simulink library "SUB_L4_Task_10ms_SUB_STEERCTRL"  (R2018a)
settings: Solver=VariableStepAuto  StartTime=0.0  StopTime=10.0  RelTol=1e-3
undefined symbols (not defined in the file or in its folder): Curvature_FF_Gain, DiscIntNeverNeededParam, Lateral_Control_Curvature_Limit, Lateral_Control_D, Lateral_Control_Error_Limit, Lateral_Control_Error_Rate_Limit, Lateral_Control_I, Lateral_Control_P, Lateral_Control_Rate_Limit_APV, Lateral_Control_YawRate_Limit, ptc_matlab_lib, REAX_OFFSET_APV, STANLEY_GAIN_APV, UndersteerCorection, Yaw_Rate_FF_Gain
libraries: EmE_MBD_Blockset x16, simulink x9, PTC_MBDS_LIB x3
settings Model: Creator=Chris.Balton  LastModifiedBy=Gavin.Coelho

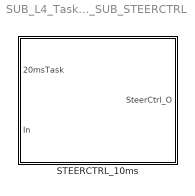
== system SUB_L4_Task_10ms_SUB_STEERCTRL ==
  STEERCTRL_10ms : Subsystem

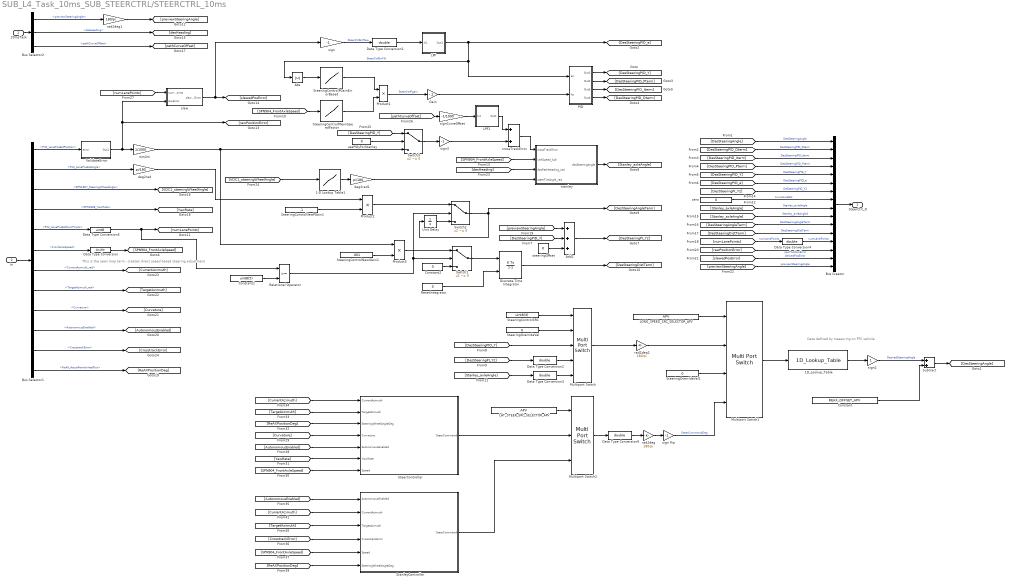
== system SUB_L4_Task_10ms_SUB_STEERCTRL/STEERCTRL_10ms ==
  note: This is the open loop term - creates direct speed based steering adjustment
  note: Data defined by measuring on PTC vehicle
  20msTask : Inport
  In : Inport  Port=2
  1-D Lookup Table1 : Lookup_n-D  NumberOfTableDimensions=1  BreakpointsForDimension1=|  Table=|  InternalRulePriority=Speed  RndMeth=Simplest  InputSameDT=on
      BreakpointsForDimension1=|
      | [-800
      | -700
      | -600
      | -500
      | -400
      | -300
      | -200
      | -100
      | 0
      | 100
      | 200
      | 300
      | 400
      | 500
      | 600
      | 700
      | 800
      | ]
      Table=|
      | [-46
      | -39.5
      | -33.5
      | -27
      | -21.5
      | -16
      | -10
      | -4.5
      | 0
      | 5.5
      | 11
      | 16
      | 21.5
      | 26
      | 31
      | 33
      | 33
      | ]
  1D_Lookup_Table : PTC_MBDS_LIB/Extras/Lookup Tables/1D_Lookup_Table  ParameterObjectName=STEERCTRL_WHEEL_ANGLE_DATA_MPV  InterpolationMethod=Linear  PTC_MBDS_BlockVersion=5.41  PTC_BlockType=PTC_MBDS_1D_Lookup_Table
      settings: SourceProductName=PACCAR Technical Center MBDS Library
      settings: AttributesFormatString=|
      | X Axis: STEERCTRL_WHEEL_ANGLE_STEP_MPV (deg)
      | Y Axis: STEERCTRL_WHEEL_ANGLE_DATA_MPV (deg)
      | Interpolation Method: Linear
  Abs : Abs
  Add2 : Sum  Inputs=+++
  Bus Creator : BusCreator  Inputs=16
  Bus Selector1 : BusSelector  OutputSignals=CAN.PX2_Lane.LanePosEst.PX2_LanePosEstPosition,CAN.PX2_Lane.LanePosEst.PX2_LanePosEstAngle,CAN.VDC2_0B.SPN1807_SteeringWheelAngle,CAN.VDC2_0B.SPN1808_YawRate,CAN.PX2_Lane.LanePosEst.PX2_LanePosEstNumPoints,CAN.EBC2_0B.FrontAxleSpeed,PIC_Bus.CurrentAzimuth_rad,PIC_Bus.TargetAzimuth_rad,PIC_Bus.Curvature,AutonomousState.AutonomousEnabled,PIC_Bus.CrosstrackError,CAN.ReAX.ReAX_ActualHandwheelPos
  Bus Selector2 : BusSelector  OutputSignals=mapping.previewSteeringAngle,mapping.desHeading,mapping.pathCurveOffset
  Constant : Constant  Value=REAX_OFFSET_APV
  Constant1 : Constant  Value=uint8(5)
  Constant2 : Constant  Value=0
  Data Type Conversion{,1..4,6} (6 alike) : DataTypeConversion  OutDataTypeStr=double
  Data Type Conversion5 : DataTypeConversion  OutDataTypeStr=uint8
  Discrete-Time Integrator : DiscreteIntegrator  ExternalReset=level  SampleTime=.01  LimitOutput=on  UpperSaturationLimit=1000  LowerSaturationLimit=-1000  ICPrevOutput=DiscIntNeverNeededParam  ICPrevScaledInput=DiscIntNeverNeededParam
  Gain : Gain  Gain=-.2
  LAT_STEER_SRC_SELECTOR_APV : EmE_MBD_Blockset/Sources/APV  conval=LAT_STEER_SRC_SELECTOR_APV
      settings: SourceProductName=PACCAR EmE MBD Blockset
  LONG_SPEED_SRC_SELECTOR_APV : EmE_MBD_Blockset/Sources/APV  conval=LONG_SPEED_SRC_SELECTOR_APV
      settings: SourceProductName=PACCAR EmE MBD Blockset
  LPF : Subsystem
  LPF1 : Subsystem
  Multiport Switch : MultiPortSwitch  DataPortOrder=Zero-based contiguous  Inputs=4  zeroidx=on
  Multiport Switch1 : MultiPortSwitch  DataPortOrder=Specify indices  DataPortIndices={ENUM_LONG_SPEED_DEMAND_SOURCE_T.GPS_PATH,ENUM_LONG_SPEED_DEMAND_SOURCE_T.OVERRIDE,ENUM_LONG_SPEED_DEMAND_SOURCE_T.WAYPOINTS}  DiagnosticForDefault=None
  Multiport Switch2 : MultiPortSwitch  DataPortOrder=Specify indices  DataPortIndices={ENUM_LAT_STEER_SOURCE_T.PIC_HARIS,ENUM_LAT_STEER_SOURCE_T.PIC_STANLEY}  DiagnosticForDefault=None
  PID : Subsystem
  Product1 : Product
  Product2 : Product
  Product3 : Product
  Relational Operator : RelationalOperator  OutDataTypeStr=boolean  RndMeth=Nearest
  ResetIntegrator : Constant  Value=0
  StanleyController : Subsystem
  SteerController : Subsystem
  SteeringControlNewIGain1 : Constant  Value=.001
  SteeringControlNewPGain1 : Constant  Value=.1
  SteeringControlPGainErrorBased : Lookup_n-D  NumberOfTableDimensions=1  BreakpointsForDimension1=[0 .005 .01 .02 .035 .05 .1 .2 .3 .5]  Table=[100 250 300 400 500 500 400 400 400 200]  InternalRulePriority=Speed  RndMeth=Simplest  InputSameDT=on
  SteeringControlPGainSpeedFactor : Lookup_n-D  NumberOfTableDimensions=1  BreakpointsForDimension1=[10 20 30 40 50 60 70 80 90]  Table=[.5 .5 .43 .38 .3 .2 .2 .2 .2]  InternalRulePriority=Speed  RndMeth=Simplest  InputSameDT=on
  SteeringControlSRC : Constant  Value=uint8(3)
  SteeringOverrideVal : Constant  Value=0
  SteeringOverrideVal1 : Constant  Value=0
  Subtract : Sum  InputSameDT=on
  Switch1 : Switch  Criteria=u2 ~= 0
  Switch2 : Switch  Criteria=u2 ~= 0
  Switch3 : Switch  Criteria=u2 ~= 0
  Unit Delay : UnitDelay  SampleTime=-1
  ValidateError : Subsystem
  crossTrackError : Sum
  deg2rad : Gain  Gain=pi/180
  deg2rad1 : Gain  Gain=pi/180
  mm2m : Gain  Gain=1/1000  OutDataTypeStr=double
  rad2deg : Gain  Gain=180/pi
  rad2deg1 : Gain  Gain=180/pi
  rad2deg2 : Gain  Gain=180/pi
  sign : Gain  Gain=-1
  sign flip : Gain  Gain=-1
  sign2 : Gain
  sign3 : Gain  Gain=-1
  signCurveOffset : Gain  Gain=-1/1000
  slew : Subsystem
  stanley : Subsystem
  steeringOffset : Constant  Value=0
  usePIDyForStanley : Constant  Value=0
  zero : Constant  Value=0
  SteerCtrl_O : Outport
  wires:
  [CrosstrackError] -> StanleyController/4(CriosstrackError)
  Bus Selector1/11 -> [CrosstrackError]  "<CrosstrackError>"
  Bus Selector1/12 -> [ReAXPositionDeg]  "<ReAX_ActualHandwheelPos>"
  Bus Selector1/9 -> [Curvature]  "<Curvature>"
  [Curvature] -> SteerController/4(Curvature)
  [AutonomousEnabled] -> SteerController/5(AutonomousEnabled)
  [YawRate] -> SteerController/6(YawRate)
  Bus Selector1/8 -> [TargetAzimuth]  "<TargetAzimuth_rad>"
  Bus Selector1/7 -> [CurrentAzimuth]  "<CurrentAzimuth_rad>"
  Bus Selector1/4 -> [YawRate]  "<SPN1808_YawRate>"
  rad2deg/1 -> sign flip/1
  sign flip/1 -> Multiport Switch1/4  "SteerCommandDeg"
  Bus Selector1/2 -> deg2rad/1  "<PX2_LanePosEstAngle>"
  1-D Lookup Table1/1 -> deg2rad1/1
  sign/1 -> Data Type Conversion1/1  "SteerCtrlErrRaw"
  Relational Operator/1 -> Switch1/2, Switch2/2
  20msTask/1 -> Bus Selector2/1
  Switch2/1 -> Unit Delay/1, [DesSteeringAngleTerm]
  [DesSteeringPID_Iterm] -> Bus Creator/3  "DesSteeringPID_Iterm"
  mm2m/1 -> Product3/1, Switch3/3
  LPF/1(Out1) -> [DesSteeringPID_e], Abs/1, PID/1(err)  "SteerCtrlErrFilt"
  SteeringControlPGainErrorBased/1 -> Product1/1
  PID/3(Out3) -> [DesSteeringPID_Iterm]
  deg2rad/1 -> Product2/1
  [Stanley_axleAngle] -> Bus Creator/10  "Stanley_axleAngle2"
  [VDC1_steeringWheelAngle] -> 1-D Lookup Table1/1
  Product3/1 -> Switch1/1
  Bus Selector1/5 -> Data Type Conversion5/1  "<PX2_LanePosEstNumPoints>"
  [DesSteeringPID_Y] -> Bus Creator/5  "DesSteeringPID_Y"
  [DesSteeringPID_e] -> Bus Creator/6  "DesSteeringPID_e"
  [DesSteeringPID_Pterm] -> Bus Creator/4  "DesSteeringPID_Pterm"
  Unit Delay/1 -> Switch2/3
  Data Type Conversion/1 -> [SPN904_FrontAxleSpeed]
  Add2/1 -> [DesSteeringPI_Y2]
  SteerController/1(SteerCommand) -> Multiport Switch2/2
  SteeringControlNewPGain1/1 -> Product2/2
  Product1/1 -> Gain/1  "SteerCtrlPgain"
  Gain/1 -> PID/2(kp)
  ResetIntegrator/1 -> Discrete-Time Integrator/2
  Constant1/1 -> Relational Operator/2
  zero/1 -> Bus Creator/8  "CurvatureEst"
  [DesSteeringAngleTerm] -> Bus Creator/11  "DesSteeringAngleTerm"
  deg2rad1/1 -> stanley/4(steerTireAngle_rad)
  Data Type Conversion4/1 -> Bus Creator/13  "numLanePoints"
  Data Type Conversion3/1 -> Multiport Switch/5
  [DesSteeringPI_Y2] -> Data Type Conversion2/1
  [pathCurveOffset] -> signCurveOffset/1
  Product2/1 -> Switch2/1
  SteeringControlSRC/1 -> Multiport Switch/1
  Discrete-Time Integrator/1 -> [DesSteeringDistTerm]
  [Stanley_axleAngle] -> Data Type Conversion3/1
  [Stanley_axleAngle] -> Bus Creator/9  "Stanley_axleAngle"
  [DesSteeringPI_Y2] -> Bus Creator/7  "DeSteeringPID_Y2"
  Bus Selector2/1 -> rad2deg1/1  "<previewSteeringAngle>"
  [DesSteeringPID_Dterm] -> Bus Creator/2  "DesSteeringPID_Dterm"
  [DesSteeringDistTerm] -> Bus Creator/12  "DesSteeringDistTerm"
  Switch1/1 -> Discrete-Time Integrator/1
  LONG_SPEED_SRC_SELECTOR_APV/1 -> Multiport Switch1/1
  Constant2/1 -> Switch1/3
  [DesSteeringPID_Y] -> Add2/2
  Abs/1 -> SteeringControlPGainErrorBased/1
  In/1 -> Bus Selector1/1
  PID/1(Out1) -> [DesSteeringPID_Y]
  PID/4(Out4) -> [DesSteeringPID_Dterm]
  rad2deg1/1 -> [previewSteeringAngle]
  [DesSteeringPID_Y] -> Switch3/1
  steeringOffset/1 -> Add2/3
  [numLanePoints] -> Data Type Conversion4/1  "numLanePoints"
  Bus Selector1/1 -> ValidateError/1(error)  "<PX2_LanePosEstPosition>"
  Data Type Conversion1/1 -> LPF/1(In1)
  [numLanePoints] -> slew/1(numLanePoints)
  stanley/1(desSteeringAngle) -> [Stanley_axleAngle]
  signCurveOffset/1 -> LPF1/1(In1)
  [SPN904_FrontAxleSpeed] -> SteeringControlPGainSpeedFactor/1
  [DesSteeringPID_Y] -> Multiport Switch/3
  crossTrackError/1 -> stanley/1(crossTrackError)
  Switch3/1 -> sign3/1
  [slewedPosError] -> Bus Creator/15  "slewedPosError"
  Multiport Switch1/1 -> 1D_Lookup_Table/1
  Data Type Conversion6/1 -> rad2deg/1
  Bus Selector1/3 -> [VDC1_steeringWheelAngle]  "<SPN1807_SteeringWheelAngle>"
  sign2/1 -> Subtract/1  "DesiredSteeringAngle"
  SteeringOverrideVal1/1 -> Multiport Switch1/3
  [rawPositionError] -> Bus Creator/14  "rawPositionError"
  slew/1(slewedError) -> [slewedPosError], sign/1
  Multiport Switch/1 -> rad2deg2/1
  Bus Selector2/3 -> [pathCurveOffset]  "<pathCurveOffset>"
  Data Type Conversion2/1 -> Multiport Switch/4
  PID/2(Out2) -> [DesSteeringPID_Pterm]
  sign3/1 -> crossTrackError/2
  [previewSteeringAngle] -> Add2/1
  Data Type Conversion5/1 -> [numLanePoints], Relational Operator/1
  SteeringControlPGainSpeedFactor/1 -> Product1/2
  1D_Lookup_Table/1 -> sign2/1
  [desHeading] -> stanley/3(desPathHeading_rad)
  [DesSteeringAngle] -> Bus Creator/1  "DesSteeringAngle"
  Bus Creator/1 -> SteerCtrl_O/1
  ValidateError/1(Out1) -> mm2m/1, slew/2(rawError), [rawPositionError]
  rad2deg2/1 -> Multiport Switch1/2
  usePIDyForStanley/1 -> Switch3/2
  Bus Selector2/2 -> [desHeading]  "<desHeading>"
  SteeringControlNewIGain1/1 -> Product3/2
  Bus Selector1/6 -> Data Type Conversion/1  "<FrontAxleSpeed>"
  LPF1/1(Out1) -> crossTrackError/1
  [previewSteeringAngle] -> Bus Creator/16  "previewSteeringAngle"
  Bus Selector1/10 -> [AutonomousEnabled]  "<AutonomousEnabled>"
  [SPN904_FrontAxleSpeed] -> stanley/2(vehSpeed_kph)
  SteeringOverrideVal/1 -> Multiport Switch/2
  [SPN904_FrontAxleSpeed] -> SteerController/7(Speed)
  Subtract/1 -> [DesSteeringAngle]
  Constant/1 -> Subtract/2
  [ReAXPositionDeg] -> SteerController/3(SteeringWheelAngleDeg)
  [TargetAzimuth] -> SteerController/2(TargetAzimuth)
  [CurrentAzimuth] -> SteerController/1(CurrentAzimuth)
  [ReAXPositionDeg] -> StanleyController/6(SteeringWheelAngleDeg)
  [TargetAzimuth] -> StanleyController/3(TargetAzimuth)
  [CurrentAzimuth] -> StanleyController/2(CurrentAzimuth)
  [AutonomousEnabled] -> StanleyController/1(AutonomousEnabled)
  [SPN904_FrontAxleSpeed] -> StanleyController/5(Speed)
  Multiport Switch2/1 -> Data Type Conversion6/1
  StanleyController/1(SteerCommand) -> Multiport Switch2/3
  LAT_STEER_SRC_SELECTOR_APV/1 -> Multiport Switch2/1

== system SUB_L4_Task_10ms_SUB_STEERCTRL/STEERCTRL_10ms/LPF ==
  In1 : Inport
  Constant : Constant  Value=0.1
  Constant1 : Constant  Value=ptc_matlab_lib.get_system_sample_time()
  LowpassT_RE : PTC_MBDS_LIB/MBDS Standard Library/Extended Operations/Filters/LowpassT_RE  dT_Enabled=on  dT=ptc_matlab_lib.get_system_sample_time()  E_Enabled=off  R_Enabled=off  IV_Enabled=off  IV=0  PTC_MBDS_BlockVersion=5.41  PTC_BlockType=PTC_MBDS_LowpassT_RE
      settings: AttributesFormatString=IV = %<IV>  SourceProductName=PACCAR Technical Center MBDS Library
  Out1 : Outport
  wires:
  Constant1/1 -> LowpassT_RE/2
  Constant/1 -> LowpassT_RE/1
  LowpassT_RE/1 -> Out1/1
  In1/1 -> LowpassT_RE/3

== system SUB_L4_Task_10ms_SUB_STEERCTRL/STEERCTRL_10ms/LPF1 ==
  In1 : Inport
  Constant : Constant  Value=2.0
  Constant1 : Constant  Value=0.01
  Data Type Conversion : DataTypeConversion  OutDataTypeStr=boolean  SaturateOnIntegerOverflow=on
  LowpassT_RE : PTC_MBDS_LIB/MBDS Standard Library/Extended Operations/Filters/LowpassT_RE  dT_Enabled=on  dT=ptc_matlab_lib.get_system_sample_time()  E_Enabled=off  R_Enabled=on  IV_Enabled=off  IV=0  PTC_MBDS_BlockVersion=5.41  PTC_BlockType=PTC_MBDS_LowpassT_RE
      settings: AttributesFormatString=IV = %<IV>  SourceProductName=PACCAR Technical Center MBDS Library
  Step : Step  Time=ptc_matlab_lib.get_system_sample_time()  Before=1  After=0
  Out1 : Outport
  wires:
  In1/1 -> LowpassT_RE/3
  LowpassT_RE/1 -> Out1/1
  Constant/1 -> LowpassT_RE/1
  Step/1 -> Data Type Conversion/1
  Data Type Conversion/1 -> LowpassT_RE/4
  Constant1/1 -> LowpassT_RE/2

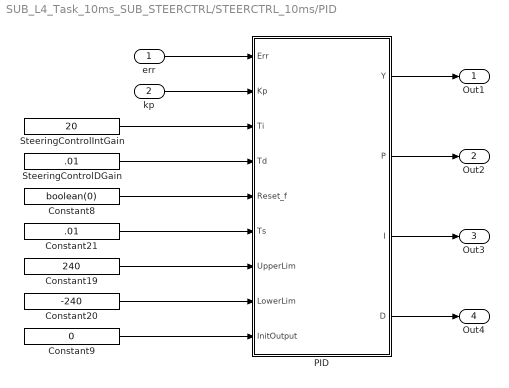
== system SUB_L4_Task_10ms_SUB_STEERCTRL/STEERCTRL_10ms/PID ==
  err : Inport
  kp : Inport  Port=2
  Constant19 : Constant  Value=240
  Constant20 : Constant  Value=-240
  Constant21 : Constant  Value=.01
  Constant8 : Constant  Value=boolean(0)
  Constant9 : Constant  Value=0
  PID : Subsystem
  SteeringControlDGain : Constant  Value=.01
  SteeringControlIntGain : Constant  Value=20
  Out1 : Outport
  Out2 : Outport  Port=2
  Out3 : Outport  Port=3
  Out4 : Outport  Port=4
  wires:
  err/1 -> PID/1(Err)
  kp/1 -> PID/2(Kp)
  Constant9/1 -> PID/9(InitOutput)
  Constant20/1 -> PID/8(LowerLim)
  Constant19/1 -> PID/7(UpperLim)
  Constant21/1 -> PID/6(Ts)
  Constant8/1 -> PID/5(Reset_f)
  PID/3(I) -> Out3/1
  PID/4(D) -> Out4/1
  PID/2(P) -> Out2/1
  PID/1(Y) -> Out1/1
  SteeringControlIntGain/1 -> PID/3(Ti)
  SteeringControlDGain/1 -> PID/4(Td)

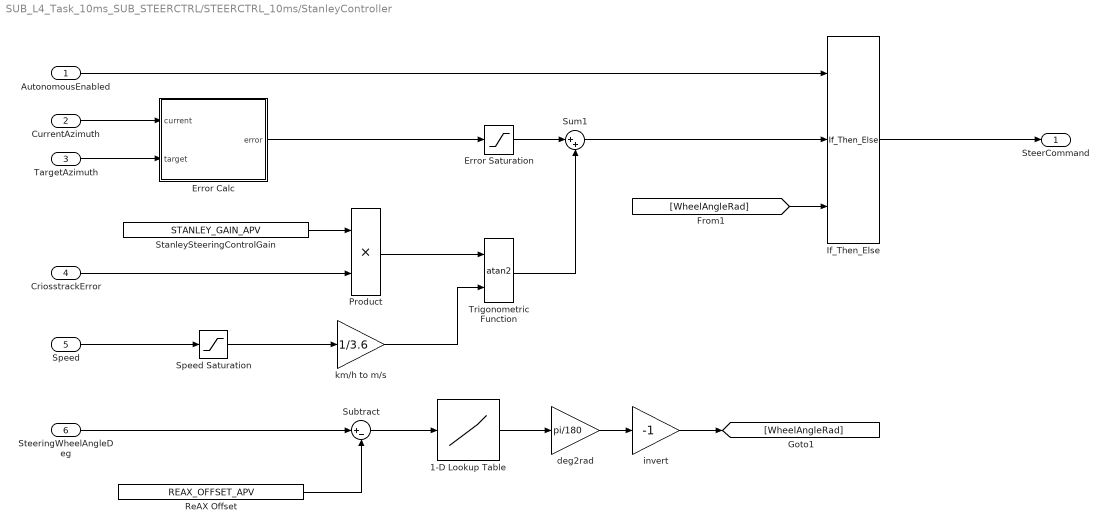
== system SUB_L4_Task_10ms_SUB_STEERCTRL/STEERCTRL_10ms/StanleyController ==
  AutonomousEnabled : Inport
  CurrentAzimuth : Inport  Port=2
  TargetAzimuth : Inport  Port=3
  CriosstrackError : Inport  Port=4
  Speed : Inport  Port=5
  SteeringWheelAngleDeg : Inport  Port=6
  1-D Lookup Table : Lookup_n-D  NumberOfTableDimensions=1  BreakpointsForDimension1=|  Table=|  InternalRulePriority=Speed  RndMeth=Simplest  InputSameDT=on
      BreakpointsForDimension1=|
      | [-800.0200195
      | -780.0289917
      | -760.0339966
      | -740
      | -720
      | -700.0040283
      | -680
      | -660.0139771
      | -640.0189819
      | -620.0239868
      | -600.0200195
      | -580.0339966
      | -560.0390015
      | -540
      | -520.0040283
      | -500.0090027
      | -480.0140076
      | -460.0190125
      | -440.0239868
      | -420.019989
      | -400.0339966
      | -380.0390015
      | -360
      | -340.0039978
      | -320.0090027
      | -300.0140076
      | -280.0190125
      | -260.0239868
      | -240.029007
      | -220.0339966
      | -200.0390015
      | -180
      | -160.0039978
      | -140.0090027
      | -120.0139999
      | -100.0189972
      | -80.02400208
      | -60.02899933
      | -40.0340004
      | 0.52700001
      | 29.96999931
      | 50.00899887
      | 69.95999908
      | 89.94999695
      | 109.9950027
      | 129.9900055
      | 149.9850006
      | 170.0240021
      | 189.9750061
      | 209.9700012
      | 229.9649963
      | 249.9600067
      | 270
      | 289.9949951
      | 309.9899902
      | 329.9849854
      | 349.980011
      | 369.9750061
      | 390.0140076
      | 410.0090027
      | 450
      | 470.0299988
      | 489.9899902
      | 509.9849854
      | 529.9799805
      | 549.9749756
      | 569.9699707
      | 589.9650269
      | 610.2199707
      | 630
      | 650.25
      | 670]
      Table=|
      | [-46
      | -44.5
      | -43
      | -42
      | -40
      | -39
      | -37.5
      | -36.5
      | -35
      | -34
      | -33
      | -31.5
      | -30.5
      | -29
      | -28
      | -26.5
      | -25.5
      | -24.5
      | -23.5
      | -22
      | -21
      | -20
      | -19
      | -17.5
      | -16.5
      | -15.5
      | -14
      | -13
      | -12
      | -11
      | -10
      | -8.5
      | -7.5
      | -6.5
      | -5
      | -4
      | -3
      | -2
      | -1
      | 0
      | 1
      | 3
      | 4
      | 5
      | 6
      | 7
      | 8
      | 9
      | 10
      | 11
      | 12
      | 13
      | 14
      | 15
      | 16
      | 17
      | 18.5
      | 19.5
      | 20.5
      | 21.5
      | 23.5
      | 24.5
      | 25.5
      | 26.5
      | 27.5
      | 28.5
      | 29
      | 30
      | 31
      | 31.5
      | 32.5
      | 33]
  Error Saturation : Saturate  UpperLimit=pi/2  LowerLimit=-pi/2
  Error Calc : MATLAB Function  TreatAsAtomicUnit=on
  If_Then_Else : EmE_MBD_Blockset/Signal Routing/If_Then_Else
      settings: SourceProductName=PACCAR EmE MBD Blockset
  Product : Product
  ReAX Offset : Constant  Value=REAX_OFFSET_APV
  Speed Saturation : Saturate  UpperLimit=255  LowerLimit=7.5
  StanleySteeringControlGain : Constant  Value=STANLEY_GAIN_APV
  Subtract : Sum  Inputs=|+-  InputSameDT=on
  Sum1 : Sum  Inputs=|++
  Trigonometric Function : Trigonometry  Operator=atan2
  deg2rad : Gain  Gain=pi/180
  invert : Gain  Gain=-1
  km/h to m/s : Gain  Gain=1/3.6  OutDataTypeStr=double
  SteerCommand : Outport
  wires:
  Error Calc/1(error) -> Error Saturation/1
  SteeringWheelAngleDeg/1 -> Subtract/1
  If_Then_Else/1 -> SteerCommand/1
  TargetAzimuth/1 -> Error Calc/2(target)
  [WheelAngleRad] -> If_Then_Else/3
  AutonomousEnabled/1 -> If_Then_Else/1
  CurrentAzimuth/1 -> Error Calc/1(current)
  1-D Lookup Table/1 -> deg2rad/1
  deg2rad/1 -> invert/1
  Sum1/1 -> If_Then_Else/2
  Subtract/1 -> 1-D Lookup Table/1
  ReAX Offset/1 -> Subtract/2
  invert/1 -> [WheelAngleRad]
  CriosstrackError/1 -> Product/2
  km/h to m/s/1 -> Trigonometric Function/2
  Product/1 -> Trigonometric Function/1
  Speed/1 -> Speed Saturation/1
  Speed Saturation/1 -> km/h to m/s/1
  Trigonometric Function/1 -> Sum1/2
  Error Saturation/1 -> Sum1/1
  StanleySteeringControlGain/1 -> Product/1

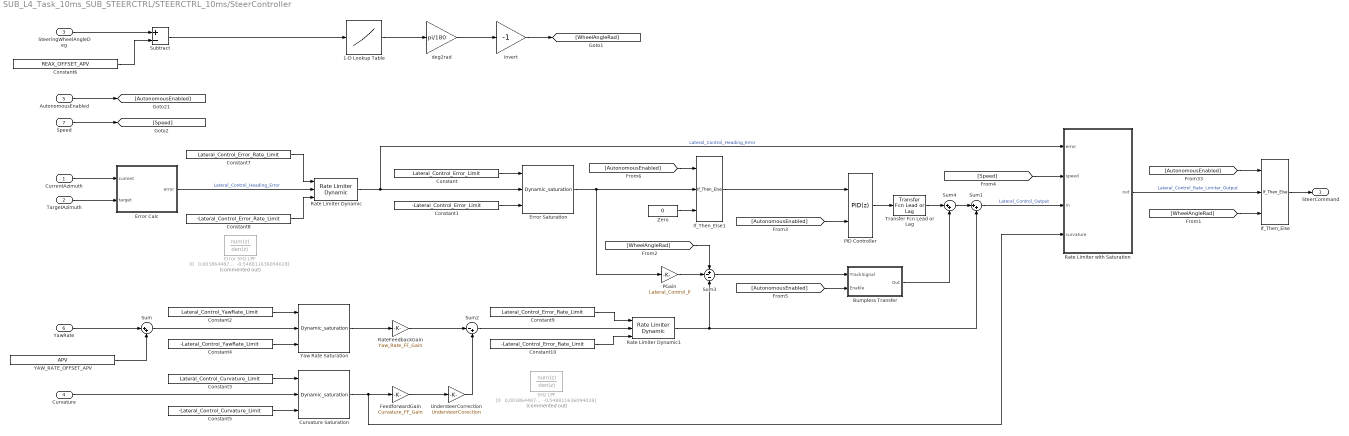
== system SUB_L4_Task_10ms_SUB_STEERCTRL/STEERCTRL_10ms/SteerController ==
  CurrentAzimuth : Inport
  TargetAzimuth : Inport  Port=2
  SteeringWheelAngleDeg : Inport  Port=3
  Curvature : Inport  Port=4
  AutonomousEnabled : Inport  Port=5
  YawRate : Inport  Port=6
  Speed : Inport  Port=7
  1-D Lookup Table : Lookup_n-D  NumberOfTableDimensions=1  BreakpointsForDimension1=|  Table=|  InternalRulePriority=Speed  RndMeth=Simplest  InputSameDT=on
      BreakpointsForDimension1=|
      | [-800.0200195
      | -780.0289917
      | -760.0339966
      | -740
      | -720
      | -700.0040283
      | -680
      | -660.0139771
      | -640.0189819
      | -620.0239868
      | -600.0200195
      | -580.0339966
      | -560.0390015
      | -540
      | -520.0040283
      | -500.0090027
      | -480.0140076
      | -460.0190125
      | -440.0239868
      | -420.019989
      | -400.0339966
      | -380.0390015
      | -360
      | -340.0039978
      | -320.0090027
      | -300.0140076
      | -280.0190125
      | -260.0239868
      | -240.029007
      | -220.0339966
      | -200.0390015
      | -180
      | -160.0039978
      | -140.0090027
      | -120.0139999
      | -100.0189972
      | -80.02400208
      | -60.02899933
      | -40.0340004
      | 0.52700001
      | 29.96999931
      | 50.00899887
      | 69.95999908
      | 89.94999695
      | 109.9950027
      | 129.9900055
      | 149.9850006
      | 170.0240021
      | 189.9750061
      | 209.9700012
      | 229.9649963
      | 249.9600067
      | 270
      | 289.9949951
      | 309.9899902
      | 329.9849854
      | 349.980011
      | 369.9750061
      | 390.0140076
      | 410.0090027
      | 450
      | 470.0299988
      | 489.9899902
      | 509.9849854
      | 529.9799805
      | 549.9749756
      | 569.9699707
      | 589.9650269
      | 610.2199707
      | 630
      | 650.25
      | 670]
      Table=|
      | [-46
      | -44.5
      | -43
      | -42
      | -40
      | -39
      | -37.5
      | -36.5
      | -35
      | -34
      | -33
      | -31.5
      | -30.5
      | -29
      | -28
      | -26.5
      | -25.5
      | -24.5
      | -23.5
      | -22
      | -21
      | -20
      | -19
      | -17.5
      | -16.5
      | -15.5
      | -14
      | -13
      | -12
      | -11
      | -10
      | -8.5
      | -7.5
      | -6.5
      | -5
      | -4
      | -3
      | -2
      | -1
      | 0
      | 1
      | 3
      | 4
      | 5
      | 6
      | 7
      | 8
      | 9
      | 10
      | 11
      | 12
      | 13
      | 14
      | 15
      | 16
      | 17
      | 18.5
      | 19.5
      | 20.5
      | 21.5
      | 23.5
      | 24.5
      | 25.5
      | 26.5
      | 27.5
      | 28.5
      | 29
      | 30
      | 31
      | 31.5
      | 32.5
      | 33]
  5Hz LPF : DiscreteTransferFcn  Commented=on  Numerator="[0   0.003864487551074   0.013274721856995   0.002862882791433]"  Denominator="[1.000000000000000  -2.404462450768444   1.973276179061975  -0.548811636094028]"  SampleTime=0.01
  Bumpless Transfer : Subsystem
  Constant : Constant  Value=Lateral_Control_Error_Limit
  Constant1 : Constant  Value=-Lateral_Control_Error_Limit
  Constant10 : Constant  Value=-Lateral_Control_Error_Rate_Limit
  Constant2 : Constant  Value=Lateral_Control_YawRate_Limit
  Constant3 : Constant  Value=Lateral_Control_Curvature_Limit
  Constant4 : Constant  Value=-Lateral_Control_YawRate_Limit
  Constant5 : Constant  Value=-Lateral_Control_Curvature_Limit
  Constant6 : Constant  Value=REAX_OFFSET_APV
  Constant7 : Constant  Value=Lateral_Control_Error_Rate_Limit
  Constant8 : Constant  Value=-Lateral_Control_Error_Rate_Limit
  Constant9 : Constant  Value=Lateral_Control_Error_Rate_Limit
  Curvature Saturation : EmE_MBD_Blockset/Discontinuities/Dynamic_saturation
      settings: SourceProductName=PACCAR EmE MBD Blockset
  Error 5Hz LPF : DiscreteTransferFcn  Commented=on  Numerator="[0   0.003864487551074   0.013274721856995   0.002862882791433]"  Denominator="[1.000000000000000  -2.404462450768444   1.973276179061975  -0.548811636094028]"  SampleTime=0.01
  Error Calc : MATLAB Function  TreatAsAtomicUnit=on
  Error Saturation : EmE_MBD_Blockset/Discontinuities/Dynamic_saturation
      settings: SourceProductName=PACCAR EmE MBD Blockset
  FeedforwardGain : Gain  Gain=Curvature_FF_Gain
  If_Then_Else : EmE_MBD_Blockset/Signal Routing/If_Then_Else
      settings: SourceProductName=PACCAR EmE MBD Blockset
  If_Then_Else1 : EmE_MBD_Blockset/Signal Routing/If_Then_Else
      settings: SourceProductName=PACCAR EmE MBD Blockset
  PGain : Gain  Gain=Lateral_Control_P
  PID Controller : simulink/Continuous/PID Controller  Controller=PID  TimeDomain=Discrete-time  SampleTime=-1  IntegratorMethod=Forward Euler  FilterMethod=Forward Euler  Form=Parallel  UseFilter=on  ControllerParametersSource=internal  P=Lateral_Control_P  I=Lateral_Control_I  D=Lateral_Control_D  N=20  InitialConditionSource=internal  InitialConditionForIntegrator=0  InitialConditionForFilter=0  ExternalReset=rising  LimitOutput=on  UpperSaturationLimit=0.2  LowerSaturationLimit=-0.2  LinearizeAsGain=on  AntiWindupMode=none  Kb=1  TrackingMode=off  Kt=1  PParamMin=[]  PParamMax=[]  IParamMin=[]  IParamMax=[]  DParamMin=[]  DParamMax=[]  NParamMin=[]  NParamMax=[]  KbParamMin=[]  KbParamMax=[]  KtParamMin=[]  KtParamMax=[]  POutMin=[]  POutMax=[]  IOutMin=[]  IOutMax=[]  DOutMin=[]  DOutMax=[]  NOutMin=[]  NOutMax=[]  KbOutMin=[]  KbOutMax=[]  KtOutMin=[]  KtOutMax=[]  IntegratorOutMin=[]  IntegratorOutMax=[]  FilterOutMin=[]  FilterOutMax=[]  SumOutMin=[]  SumOutMax=[]  SumI1OutMin=[]  SumI1OutMax=[]  SumI2OutMin=[]  SumI2OutMax=[]  SumI3OutMin=[]  SumI3OutMax=[]  SumDOutMin=[]  SumDOutMax=[]  SaturationOutMin=[]  SaturationOutMax=[]  IntegratorContinuousStateAttributes=''  IntegratorStateMustResolveToSignalObject=off  IntegratorRTWStateStorageClass=Auto  FilterContinuousStateAttributes=''  FilterStateMustResolveToSignalObject=off  FilterRTWStateStorageClass=Auto  DifferentiatorICPrevScaledInput=0  DifferentiatorOutMin=[]  DifferentiatorOutMax=[]  FilterDiffOutCoefMin=[]  FilterDiffOutCoefMax=[]  SumDenOutMin=[]  SumDenOutMax=[]  SumNumOutMin=[]  SumNumOutMax=[]  ReciprocalOutMin=[]  ReciprocalOutMax=[]  DivideOutMin=[]  DivideOutMax=[]  TunerSelectOption=Transfer Function Based (PID Tuner App)
  Rate Limiter Dynamic : simulink/Discontinuities/Rate Limiter Dynamic
      settings: SourceProductName=Simulink
  Rate Limiter Dynamic1 : simulink/Discontinuities/Rate Limiter Dynamic
      settings: SourceProductName=Simulink
  Rate Limiter with Saturation : Subsystem
  RateFeedbackGain : Gain  Gain=Yaw_Rate_FF_Gain
  Subtract : Sum  Inputs=+-  InputSameDT=on
  Sum : Sum  Inputs=|++
  Sum1 : Sum  Inputs=|++
  Sum2 : Sum  Inputs=|-+
  Sum3 : Sum  Inputs=+--
  Sum4 : Sum  Inputs=|++
  Transfer Fcn Lead or Lag : simulink/Discrete/Transfer Fcn Lead or Lag  PoleZ=Lateral_Control_Pole  ZeroZ=Lateral_Control_Zero  ICPrevOutput=0.0  ICPrevInput=0.0  DoSatur=off
      settings: SourceProductName=Simulink  SourceProductBaseCode=SL
  UndersteerCorrection : Gain  Gain=UndersteerCorection
  YAW_RATE_OFFSET_APV : EmE_MBD_Blockset/Sources/APV  conval=YAW_RATE_OFFSET_APV
      settings: SourceProductName=PACCAR EmE MBD Blockset
  Yaw Rate Saturation : EmE_MBD_Blockset/Discontinuities/Dynamic_saturation
      settings: SourceProductName=PACCAR EmE MBD Blockset
  Zero : Constant  Value=0
  deg2rad : Gain  Gain=pi/180
  invert : Gain  Gain=-1
  SteerCommand : Outport
  wires:
  Error Calc/1(error) -> Rate Limiter Dynamic/2  "Lateral_Control_Heading_Error"
  Sum4/1 -> Sum1/1
  Constant1/1 -> Error Saturation/3
  UndersteerCorrection/1 -> Sum2/2
  [AutonomousEnabled] -> If_Then_Else1/1
  [AutonomousEnabled] -> Bumpless Transfer/2(Enable)
  AutonomousEnabled/1 -> [AutonomousEnabled]
  Error Saturation/1 -> If_Then_Else1/2, PGain/1
  SteeringWheelAngleDeg/1 -> Subtract/1
  Bumpless Transfer/1(Out) -> Sum4/2
  PGain/1 -> Sum3/2
  If_Then_Else1/1 -> PID Controller/1
  If_Then_Else/1 -> SteerCommand/1
  TargetAzimuth/1 -> Error Calc/2(target)
  Sum3/1 -> Bumpless Transfer/1(TrackSignal)
  [WheelAngleRad] -> Sum3/1
  Speed/1 -> [Speed]
  [WheelAngleRad] -> If_Then_Else/3
  [AutonomousEnabled] -> If_Then_Else/1
  RateFeedbackGain/1 -> Sum2/1
  [AutonomousEnabled] -> PID Controller/2
  Sum2/1 -> Rate Limiter Dynamic1/2
  Zero/1 -> If_Then_Else1/3
  [Speed] -> Rate Limiter with Saturation/2(speed)
  CurrentAzimuth/1 -> Error Calc/1(current)
  Curvature Saturation/1 -> Rate Limiter with Saturation/4(curvature), FeedforwardGain/1
  Rate Limiter with Saturation/1(out) -> If_Then_Else/2  "Lateral_Control_Rate_Limiter_Output"
  FeedforwardGain/1 -> UndersteerCorrection/1
  Yaw Rate Saturation/1 -> RateFeedbackGain/1
  Rate Limiter Dynamic/1 -> Rate Limiter with Saturation/1(error), Error Saturation/2  "Lateral_Control_Heading_Error"
  Rate Limiter Dynamic1/1 -> Sum1/2, Sum3/3
  Constant/1 -> Error Saturation/1
  1-D Lookup Table/1 -> deg2rad/1
  deg2rad/1 -> invert/1
  Sum1/1 -> Rate Limiter with Saturation/3(in)  "Lateral_Control_Output"
  YawRate/1 -> Sum/1
  Curvature/1 -> Curvature Saturation/2
  Constant2/1 -> Yaw Rate Saturation/1
  Constant3/1 -> Curvature Saturation/1
  Constant4/1 -> Yaw Rate Saturation/3
  Constant5/1 -> Curvature Saturation/3
  PID Controller/1 -> Transfer Fcn Lead or Lag/1
  Transfer Fcn Lead or Lag/1 -> Sum4/1
  Subtract/1 -> 1-D Lookup Table/1
  Constant6/1 -> Subtract/2
  Constant7/1 -> Rate Limiter Dynamic/1
  Constant8/1 -> Rate Limiter Dynamic/3
  invert/1 -> [WheelAngleRad]
  Constant9/1 -> Rate Limiter Dynamic1/1
  Constant10/1 -> Rate Limiter Dynamic1/3
  Sum/1 -> Yaw Rate Saturation/2
  YAW_RATE_OFFSET_APV/1 -> Sum/2

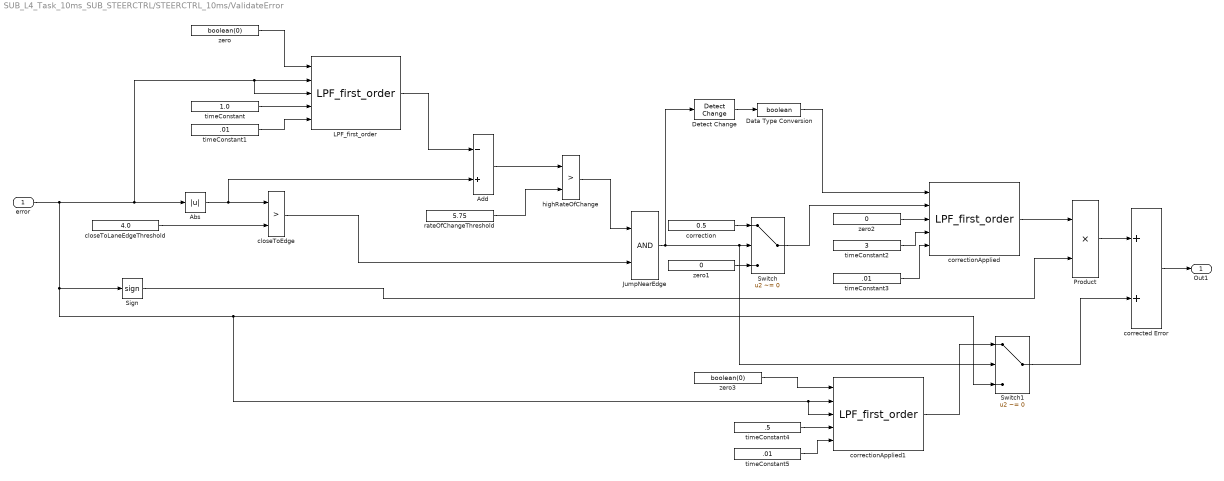
== system SUB_L4_Task_10ms_SUB_STEERCTRL/STEERCTRL_10ms/ValidateError ==
  error : Inport
  Abs : Abs
  Add : Sum  Inputs=-+
  Data Type Conversion : DataTypeConversion  OutDataTypeStr=boolean
  Detect Change : simulink/Logic and Bit Operations/Detect Change  vinit=0  InputProcessing=Inherited  OutDataTypeStr=boolean
  JumpNearEdge : Logic  AllPortsSameDT=off  OutDataTypeStr=boolean
  LPF_first_order : EmE_MBD_Blockset/Discrete/LPF_first_order
      settings: SourceProductName=PACCAR EmE MBD Blockset
  Product : Product
  Sign : Signum
  Switch : Switch  Criteria=u2 ~= 0
  Switch1 : Switch  Criteria=u2 ~= 0
  closeToEdge : RelationalOperator  Operator=>  OutDataTypeStr=boolean  RndMeth=Nearest
  closeToLaneEdgeThreshold : Constant  Value=4.0
  corrected Error : Sum
  correction : Constant  Value=0.5
  correctionApplied : EmE_MBD_Blockset/Discrete/LPF_first_order
      settings: SourceProductName=PACCAR EmE MBD Blockset
  correctionApplied1 : EmE_MBD_Blockset/Discrete/LPF_first_order
      settings: SourceProductName=PACCAR EmE MBD Blockset
  highRateOfChange : RelationalOperator  Operator=>  OutDataTypeStr=boolean  RndMeth=Nearest
  rateOfChangeThreshold : Constant  Value=5.75
  timeConstant : Constant  Value=1.0
  timeConstant1 : Constant  Value=.01
  timeConstant2 : Constant  Value=3
  timeConstant3 : Constant  Value=.01
  timeConstant4 : Constant  Value=.5
  timeConstant5 : Constant  Value=.01
  zero : Constant  Value=boolean(0)
  zero1 : Constant  Value=0
  zero2 : Constant  Value=0
  zero3 : Constant  Value=boolean(0)
  Out1 : Outport
  wires:
  Switch1/1 -> corrected Error/2
  correctionApplied1/1 -> Switch1/1
  timeConstant5/1 -> correctionApplied1/5
  timeConstant4/1 -> correctionApplied1/4
  error/1 -> Abs/1, LPF_first_order/2, LPF_first_order/3, Switch1/3, correctionApplied1/2, correctionApplied1/3, Sign/1
  zero3/1 -> correctionApplied1/1
  Data Type Conversion/1 -> correctionApplied/1
  corrected Error/1 -> Out1/1
  Product/1 -> corrected Error/1
  Sign/1 -> Product/2
  correctionApplied/1 -> Product/1
  timeConstant3/1 -> correctionApplied/5
  timeConstant2/1 -> correctionApplied/4
  Switch/1 -> correctionApplied/2
  Detect Change/1 -> Data Type Conversion/1
  zero2/1 -> correctionApplied/3
  correction/1 -> Switch/1
  zero1/1 -> Switch/3
  JumpNearEdge/1 -> Switch/2, Switch1/2, Detect Change/1
  closeToEdge/1 -> JumpNearEdge/2
  highRateOfChange/1 -> JumpNearEdge/1
  rateOfChangeThreshold/1 -> highRateOfChange/2
  Add/1 -> highRateOfChange/1
  LPF_first_order/1 -> Add/1
  timeConstant1/1 -> LPF_first_order/5
  timeConstant/1 -> LPF_first_order/4
  zero/1 -> LPF_first_order/1
  closeToLaneEdgeThreshold/1 -> closeToEdge/2
  Abs/1 -> closeToEdge/1, Add/2

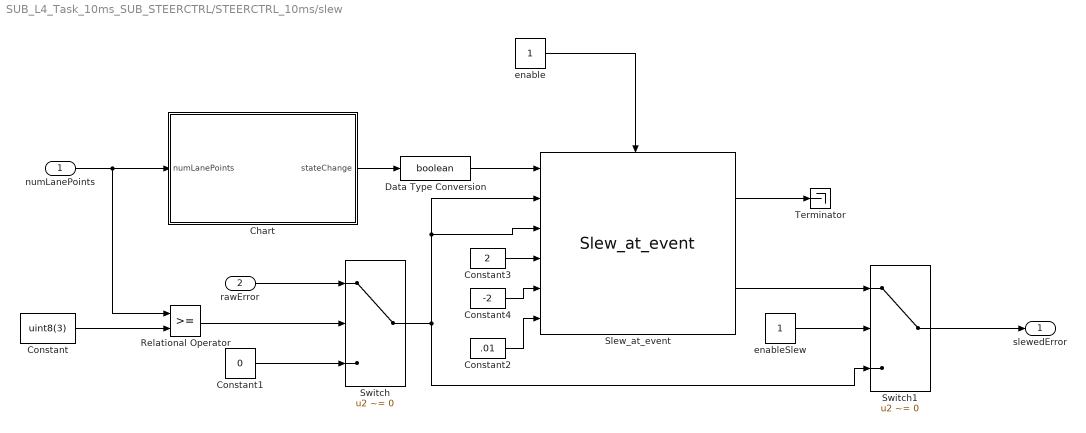
== system SUB_L4_Task_10ms_SUB_STEERCTRL/STEERCTRL_10ms/slew ==
  numLanePoints : Inport
  rawError : Inport  Port=2
  Chart : Stateflow chart  TreatAsAtomicUnit=on
  Constant : Constant  Value=uint8(3)
  Constant1 : Constant  Value=0
  Constant2 : Constant  Value=.01
  Constant3 : Constant  Value=2
  Constant4 : Constant  Value=-2
  Data Type Conversion : DataTypeConversion  OutDataTypeStr=boolean
  Relational Operator : RelationalOperator  OutDataTypeStr=boolean  RndMeth=Nearest
  Slew_at_event : EmE_MBD_Blockset/Math Operators/Slew_at_event
      settings: SourceProductName=PACCAR EmE MBD Blockset
  Switch : Switch  Criteria=u2 ~= 0
  Switch1 : Switch  Criteria=u2 ~= 0
  Terminator : Terminator
  enable : Constant
  enableSlew : Constant
  slewedError : Outport
  wires:
  enableSlew/1 -> Switch1/2
  Switch1/1 -> slewedError/1
  Data Type Conversion/1 -> Slew_at_event/1
  Constant4/1 -> Slew_at_event/5
  Constant3/1 -> Slew_at_event/4
  Constant2/1 -> Slew_at_event/6
  Switch/1 -> Slew_at_event/3, Slew_at_event/2, Switch1/3
  Relational Operator/1 -> Switch/2
  rawError/1 -> Switch/1
  Constant1/1 -> Switch/3
  Constant/1 -> Relational Operator/2
  Chart/1(stateChange) -> Data Type Conversion/1
  numLanePoints/1 -> Chart/1(numLanePoints), Relational Operator/1
  Slew_at_event/2 -> Switch1/1
  enable/1 -> Slew_at_event/Enable
  Slew_at_event/1 -> Terminator/1

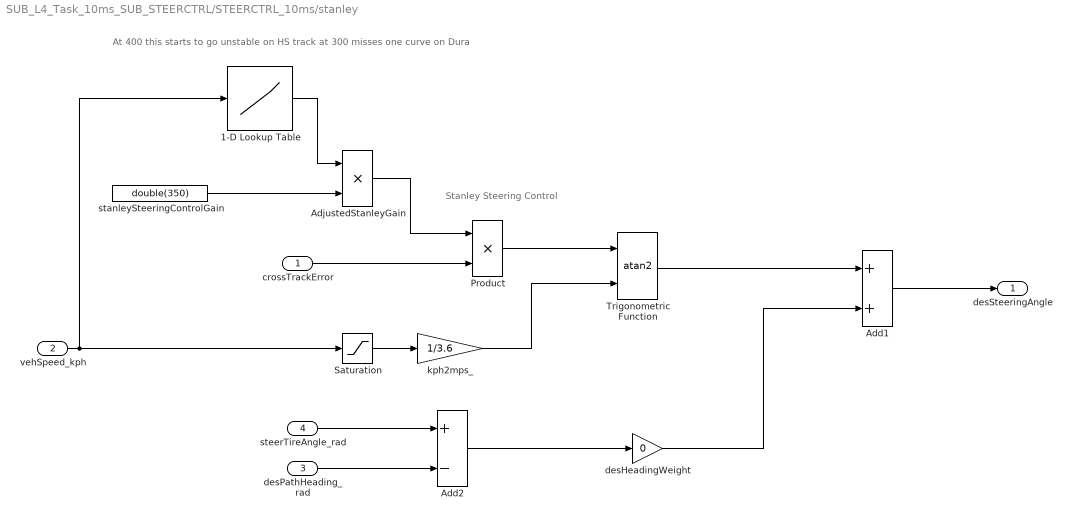
== system SUB_L4_Task_10ms_SUB_STEERCTRL/STEERCTRL_10ms/stanley ==
  note: Stanley Steering Control
  note: At 400 this starts to go unstable on HS track at 300 misses one curve on Dura
  crossTrackError : Inport
  vehSpeed_kph : Inport  Port=2
  desPathHeading_rad : Inport  Port=3
  steerTireAngle_rad : Inport  Port=4
  1-D Lookup Table : Lookup_n-D  NumberOfTableDimensions=1  BreakpointsForDimension1=[0 5 10 15 25 35 45 55 65]  Table=[.1 .5 .9 1 1 1 .9 .8 .7]  InternalRulePriority=Speed  RndMeth=Simplest  InputSameDT=on
  Add1 : Sum
  Add2 : Sum  Inputs=+-
  AdjustedStanleyGain : Product
  Product : Product
  Saturation : Saturate  UpperLimit=255  LowerLimit=7.5
  Trigonometric Function : Trigonometry  Operator=atan2
  desHeadingWeight : Gain  Gain=0
  kph2mps_ : Gain  Gain=1/3.6  OutDataTypeStr=double
  stanleySteeringControlGain : Constant  Value=double(350)
  desSteeringAngle : Outport
  wires:
  1-D Lookup Table/1 -> AdjustedStanleyGain/1
  stanleySteeringControlGain/1 -> AdjustedStanleyGain/2
  Saturation/1 -> kph2mps_/1
  desHeadingWeight/1 -> Add1/2
  desPathHeading_rad/1 -> Add2/2
  steerTireAngle_rad/1 -> Add2/1
  crossTrackError/1 -> Product/2
  Add2/1 -> desHeadingWeight/1
  Trigonometric Function/1 -> Add1/1
  vehSpeed_kph/1 -> Saturation/1, 1-D Lookup Table/1
  kph2mps_/1 -> Trigonometric Function/2
  Product/1 -> Trigonometric Function/1
  AdjustedStanleyGain/1 -> Product/1
  Add1/1 -> desSteeringAngle/1

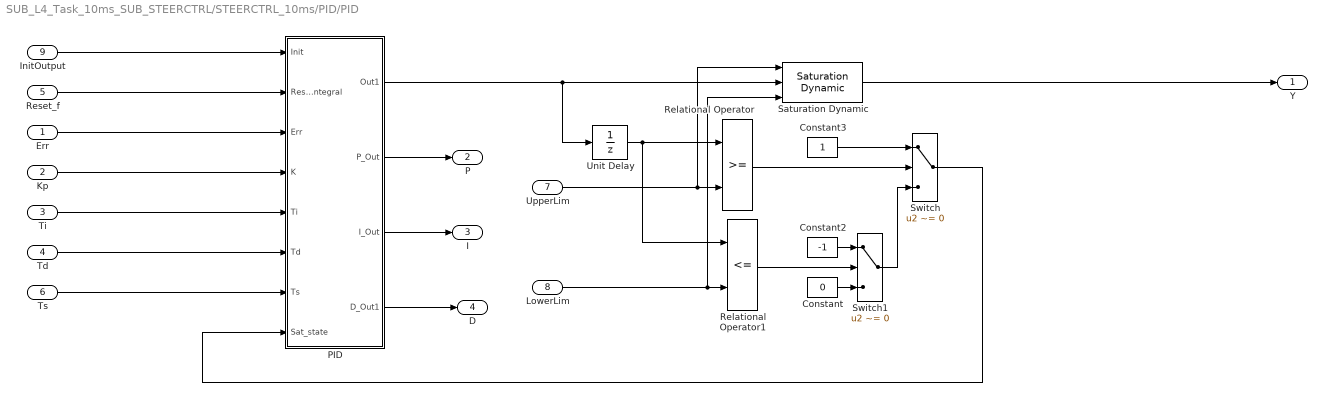
== system SUB_L4_Task_10ms_SUB_STEERCTRL/STEERCTRL_10ms/PID/PID ==
  Err : Inport
  Kp : Inport  Port=2
  Ti : Inport  Port=3
  Td : Inport  Port=4
  Reset_f : Inport  Port=5
  Ts : Inport  Port=6
  UpperLim : Inport  Port=7
  LowerLim : Inport  Port=8
  InitOutput : Inport  Port=9
  Constant : Constant  Value=0
  Constant2 : Constant  Value=-1
  Constant3 : Constant
  PID : Subsystem
  Relational Operator : RelationalOperator  OutDataTypeStr=boolean  RndMeth=Nearest
  Relational Operator1 : RelationalOperator  Operator=<=  OutDataTypeStr=boolean  RndMeth=Nearest
  Saturation Dynamic : simulink/Discontinuities/Saturation Dynamic  RequirementInfo={} %GIDa_a8a084d7_bda8_4443_856d_eb85f2a73d9b  OutMin=[]  OutMax=[]  OutDataTypeStr=Inherit: Same as second input  OutDataType=sfix(16)  OutScaling=2^-10  DoSatur=off
  Switch : Switch  Criteria=u2 ~= 0
  Switch1 : Switch  Criteria=u2 ~= 0
  Unit Delay : UnitDelay  SampleTime=-1
  Y : Outport
  P : Outport  Port=2
  I : Outport  Port=3
  D : Outport  Port=4
  wires:
  Reset_f/1 -> PID/2(Reset_Integral)
  Unit Delay/1 -> Relational Operator1/1, Relational Operator/1
  LowerLim/1 -> Relational Operator1/2, Saturation Dynamic/3
  UpperLim/1 -> Relational Operator/2, Saturation Dynamic/1
  Relational Operator/1 -> Switch/2
  Switch/1 -> PID/8(Sat_state)
  Constant3/1 -> Switch/1
  Switch1/1 -> Switch/3
  Constant2/1 -> Switch1/1
  Constant/1 -> Switch1/3
  Relational Operator1/1 -> Switch1/2
  PID/4(D_Out1) -> D/1
  PID/3(I_Out) -> I/1
  PID/2(P_Out) -> P/1
  InitOutput/1 -> PID/1(Init)
  Kp/1 -> PID/4(K)
  Ti/1 -> PID/5(Ti)
  Td/1 -> PID/6(Td)
  Ts/1 -> PID/7(Ts)
  Err/1 -> PID/3(Err)
  PID/1(Out1) -> Saturation Dynamic/2, Unit Delay/1
  Saturation Dynamic/1 -> Y/1

== system SUB_L4_Task_10ms_SUB_STEERCTRL/STEERCTRL_10ms/SteerController/Bumpless Transfer ==
  TrackSignal : Inport
  Enable : Inport  Port=2
  Discrete-Time Integrator : DiscreteIntegrator  gainval=Lateral_Control_P  ExternalReset=rising  InitialConditionSource=external  SampleTime=-1  ICPrevOutput=DiscIntNeverNeededParam  ICPrevScaledInput=DiscIntNeverNeededParam
  Gain : Gain  Gain=-1
  Out : Outport
  wires:
  Gain/1 -> Discrete-Time Integrator/1
  TrackSignal/1 -> Discrete-Time Integrator/3
  Discrete-Time Integrator/1 -> Out/1, Gain/1
  Enable/1 -> Discrete-Time Integrator/2

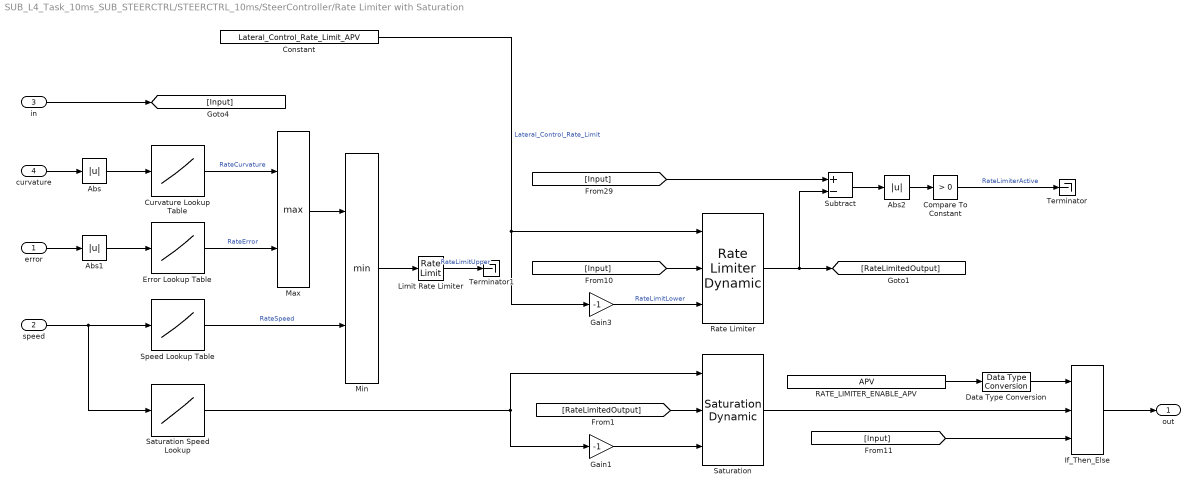
== system SUB_L4_Task_10ms_SUB_STEERCTRL/STEERCTRL_10ms/SteerController/Rate Limiter with Saturation ==
  error : Inport
  speed : Inport  Port=2
  in : Inport  Port=3
  curvature : Inport  Port=4
  Abs : Abs
  Abs1 : Abs
  Abs2 : Abs
  Compare To Constant : simulink/Logic and Bit Operations/Compare To Constant  relop=>  const=0  OutDataTypeStr=boolean
  Constant : Constant  Value=Lateral_Control_Rate_Limit_APV
  Curvature Lookup Table : Lookup_n-D  NumberOfTableDimensions=1  BreakpointsForDimension1=[0.00001,0.0001,0.1,0.2,0.5]  Table=[0.0001,0.001,0.1,0.2,1]  ExtrapMethod=Clip  UseLastTableValue=on  InternalRulePriority=Speed  RndMeth=Simplest  InputSameDT=on
  Data Type Conversion : EmE_MBD_Blockset/Signal Attributes/Data Type Conversion  OutDataTypeStr=Inherit: Inherit via back propagation
      settings: SourceProductName=PACCAR EmE MBD Blockset
  Error Lookup Table : Lookup_n-D  NumberOfTableDimensions=1  BreakpointsForDimension1=[0.001,0.01,0.1,0.5,1]  Table=[0.01,0.05,0.1,0.2,1]  ExtrapMethod=Clip  UseLastTableValue=on  InternalRulePriority=Speed  RndMeth=Simplest  InputSameDT=on
  Gain1 : Gain  Gain=-1
  Gain3 : Gain  Gain=-1
  If_Then_Else : EmE_MBD_Blockset/Signal Routing/If_Then_Else
      settings: SourceProductName=PACCAR EmE MBD Blockset
  Limit Rate Limiter : RateLimiter  RisingSlewLimit=0.5  FallingSlewLimit=-0.5  SampleTimeMode=inherited
  Max : MinMax  Function=max  Inputs=2
  Min : MinMax  Inputs=2
  RATE_LIMITER_ENABLE_APV : EmE_MBD_Blockset/Sources/APV  conval=RATE_LIMITER_ENABLE_APV
      settings: SourceProductName=PACCAR EmE MBD Blockset
  Rate Limiter : simulink/Discontinuities/Rate Limiter Dynamic
      settings: SourceProductName=Simulink
  Saturation : simulink/Discontinuities/Saturation Dynamic  OutMin=[]  OutMax=[]  OutDataTypeStr=Inherit: Same as second input  OutDataType=fixdt(1, 16)  OutScaling=2^-10  DoSatur=off
  Saturation Speed Lookup : Lookup_n-D  NumberOfTableDimensions=1  BreakpointsForDimension1=[10,20,30,50,70,100]  Table=[1,0.9,0.8,0.5,0.2,0.01]  ExtrapMethod=Clip  UseLastTableValue=on  InternalRulePriority=Speed  RndMeth=Simplest  InputSameDT=on
  Speed Lookup Table : Lookup_n-D  NumberOfTableDimensions=1  BreakpointsForDimension1=[10,20,30,50,70,100]  Table=[1,0.6,0.3,0.1,0.05,0.01]  ExtrapMethod=Clip  UseLastTableValue=on  InternalRulePriority=Speed  RndMeth=Simplest  InputSameDT=on
  Subtract : Sum  Inputs=+-
  Terminator : Terminator
  Terminator1 : Terminator
  out : Outport
  wires:
  Gain1/1 -> Saturation/3
  Saturation/1 -> If_Then_Else/2
  Saturation Speed Lookup/1 -> Gain1/1, Saturation/1
  [Input] -> If_Then_Else/3
  [Input] -> Rate Limiter/2
  in/1 -> [Input]
  [Input] -> Subtract/1
  Abs1/1 -> Error Lookup Table/1
  Compare To Constant/1 -> Terminator/1  "RateLimiterActive"
  Curvature Lookup Table/1 -> Max/1  "RateCurvature"
  Error Lookup Table/1 -> Max/2  "RateError"
  Subtract/1 -> Abs2/1
  Constant/1 -> Gain3/1, Rate Limiter/1  "Lateral_Control_Rate_Limit"
  curvature/1 -> Abs/1
  Abs/1 -> Curvature Lookup Table/1
  Abs2/1 -> Compare To Constant/1
  error/1 -> Abs1/1
  Speed Lookup Table/1 -> Min/2  "RateSpeed"
  Max/1 -> Min/1
  Rate Limiter/1 -> Subtract/2, [RateLimitedOutput]
  If_Then_Else/1 -> out/1
  RATE_LIMITER_ENABLE_APV/1 -> Data Type Conversion/1
  speed/1 -> Saturation Speed Lookup/1, Speed Lookup Table/1
  Data Type Conversion/1 -> If_Then_Else/1
  [RateLimitedOutput] -> Saturation/2
  Gain3/1 -> Rate Limiter/3  "RateLimitLower"
  Min/1 -> Limit Rate Limiter/1
  Limit Rate Limiter/1 -> Terminator1/1  "RateLimitUpper"

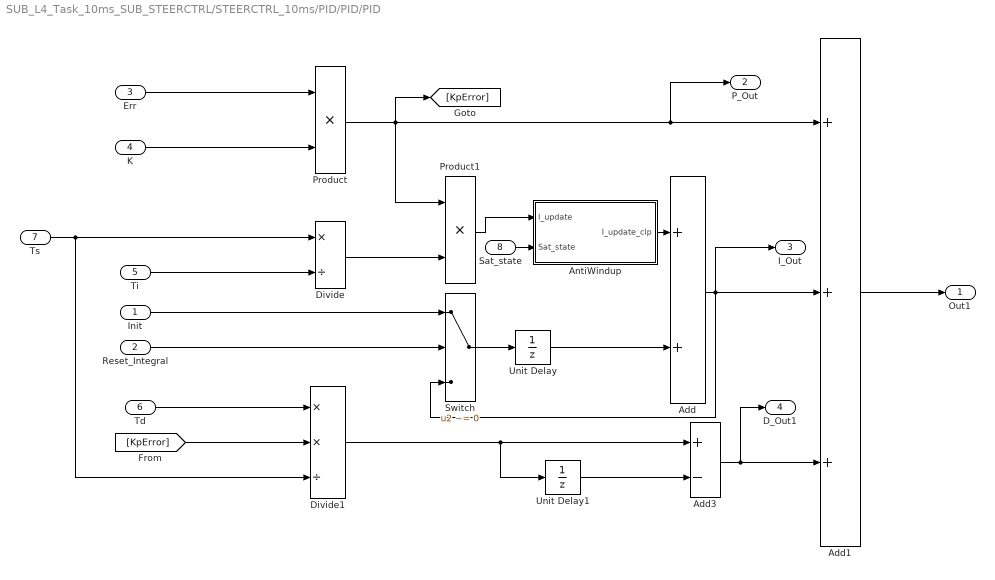
== system SUB_L4_Task_10ms_SUB_STEERCTRL/STEERCTRL_10ms/PID/PID/PID ==
  Init : Inport
  Reset_Integral : Inport  Port=2
  Err : Inport  Port=3
  K : Inport  Port=4
  Ti : Inport  Port=5
  Td : Inport  Port=6
  Ts : Inport  Port=7
  Sat_state : Inport  Port=8
  Add : Sum
  Add1 : Sum  Inputs=+++
  Add3 : Sum  Inputs=+-
  AntiWindup : Subsystem
  Divide : Product  Inputs=*/
  Divide1 : Product  Inputs=**/
  Product : Product  RndMeth=Zero
  Product1 : Product  RndMeth=Zero
  Switch : Switch  Criteria=u2 ~= 0
  Unit Delay : UnitDelay  SampleTime=-1
  Unit Delay1 : UnitDelay  SampleTime=-1
  Out1 : Outport
  P_Out : Outport  Port=2
  I_Out : Outport  Port=3
  D_Out1 : Outport  Port=4
  wires:
  Sat_state/1 -> AntiWindup/2(Sat_state)
  Product1/1 -> AntiWindup/1(I_update)
  AntiWindup/1(I_update_clp) -> Add/1
  Reset_Integral/1 -> Switch/2
  Init/1 -> Switch/1
  Err/1 -> Product/1
  K/1 -> Product/2
  Product/1 -> Product1/1, Add1/1, P_Out/1, [KpError]
  Ts/1 -> Divide1/3, Divide/1
  Ti/1 -> Divide/2
  Divide/1 -> Product1/2
  Unit Delay/1 -> Add/2
  Switch/1 -> Unit Delay/1
  Add/1 -> Switch/3, Add1/2, I_Out/1
  Add1/1 -> Out1/1
  Td/1 -> Divide1/1
  [KpError] -> Divide1/2
  Divide1/1 -> Add3/1, Unit Delay1/1
  Unit Delay1/1 -> Add3/2
  Add3/1 -> Add1/3, D_Out1/1

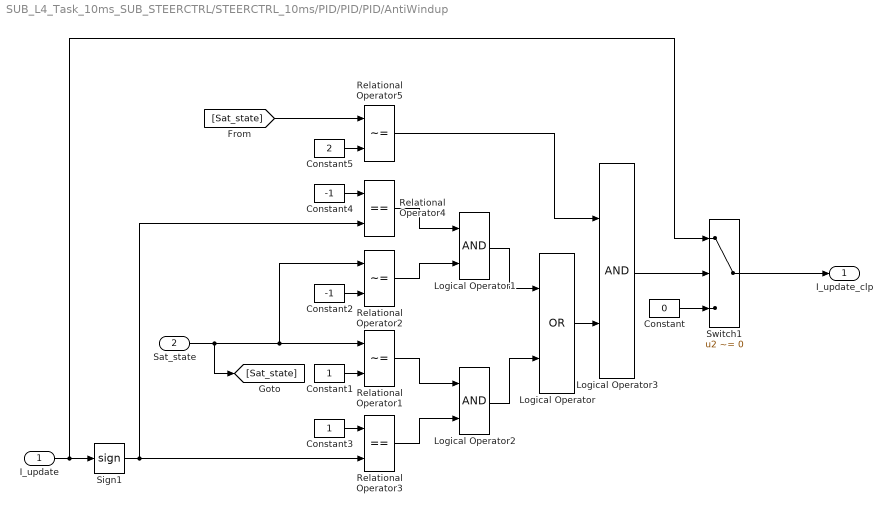
== system SUB_L4_Task_10ms_SUB_STEERCTRL/STEERCTRL_10ms/PID/PID/PID/AntiWindup ==
  I_update : Inport
  Sat_state : Inport  Port=2
  Constant : Constant  Value=0
  Constant1 : Constant
  Constant2 : Constant  Value=-1
  Constant3 : Constant
  Constant4 : Constant  Value=-1
  Constant5 : Constant  Value=2
  Logical Operator : Logic  Operator=OR  AllPortsSameDT=off  OutDataTypeStr=boolean
  Logical Operator1 : Logic  AllPortsSameDT=off  OutDataTypeStr=boolean
  Logical Operator2 : Logic  AllPortsSameDT=off  OutDataTypeStr=boolean
  Logical Operator3 : Logic  AllPortsSameDT=off  OutDataTypeStr=boolean
  Relational Operator1 : RelationalOperator  Operator=~=  OutDataTypeStr=boolean  RndMeth=Nearest
  Relational Operator2 : RelationalOperator  Operator=~=  OutDataTypeStr=boolean  RndMeth=Nearest
  Relational Operator3 : RelationalOperator  Operator===  OutDataTypeStr=boolean  RndMeth=Nearest
  Relational Operator4 : RelationalOperator  Operator===  OutDataTypeStr=boolean  RndMeth=Nearest
  Relational Operator5 : RelationalOperator  Operator=~=  OutDataTypeStr=boolean  RndMeth=Nearest
  Sign1 : Signum
  Switch1 : Switch  Criteria=u2 ~= 0
  I_update_clp : Outport
  wires:
  Relational Operator5/1 -> Logical Operator3/1
  [Sat_state] -> Relational Operator5/1
  Constant5/1 -> Relational Operator5/2
  Logical Operator/1 -> Logical Operator3/2
  Logical Operator3/1 -> Switch1/2
  Constant/1 -> Switch1/3
  Logical Operator2/1 -> Logical Operator/2
  Logical Operator1/1 -> Logical Operator/1
  Relational Operator1/1 -> Logical Operator2/1
  Relational Operator3/1 -> Logical Operator2/2
  Relational Operator4/1 -> Logical Operator1/1
  Relational Operator2/1 -> Logical Operator1/2
  Constant4/1 -> Relational Operator4/1
  Constant3/1 -> Relational Operator3/1
  Sign1/1 -> Relational Operator3/2, Relational Operator4/2
  Constant2/1 -> Relational Operator2/2
  Sat_state/1 -> [Sat_state], Relational Operator2/1, Relational Operator1/1
  Constant1/1 -> Relational Operator1/2
  I_update/1 -> Switch1/1, Sign1/1
  Switch1/1 -> I_update_clp/1

== matlab function SUB_L4_Task_10ms_SUB_STEERCTRL/STEERCTRL_10ms/StanleyController/Error Calc ==
  data: current input; target input; error output
function error = calc_error(current, target)

error = target - current;

if error < -pi
    error = error + 2*pi;
elseif error > pi
    error = error - 2*pi;
        
end

== matlab function SUB_L4_Task_10ms_SUB_STEERCTRL/STEERCTRL_10ms/SteerController/Error Calc ==
  data: current input; target input; error output
function error = calc_error(current, target)

error = target - current;

if error < -pi
    error = error + 2*pi;
elseif error > pi
        error = error - 2*pi;
        
end

== stateflow chart SUB_L4_Task_10ms_SUB_STEERCTRL/STEERCTRL_10ms/slew/Chart ==
  state init
    en:stateChange=uint8(0);
  state ZeroLanes
    en:stateChange=uint8(1);
  state OneLane
    en:stateChange=uint8(1);
  state ZeroLanes1
    en:stateChange=uint8(0);
  state OneLane1
    en:stateChange=uint8(0);
  state TwoLanes
    en:stateChange=uint8(1);
  state TwoLanes1
    en:stateChange=uint8(0);
  TwoLanes1 -> init : [numLanePoints<uint8(18)]
  (default) -> init
  init -> TwoLanes [order 2] : [numLanePoints>uint8(18)]
  OneLane1 -> init : [numLanePoints<uint8(3) ||numLanePoints>uint8(18)]
  init -> OneLane [order 3] : [numLanePoints>uint8(3)]
  ZeroLanes1 -> init : [numLanePoints>uint8(3)]
  init -> ZeroLanes [order 1] : [numLanePoints<=uint8(3)]
  ZeroLanes -> ZeroLanes1
  OneLane -> OneLane1
  TwoLanes -> TwoLanes1
  data: numLanePoints input uint8; stateChange output uint8
